simulink model "Kalman_Filter"  (R2021a)
settings: Solver=VariableStepAuto  StartTime=0.0  StopTime=10.0  RelTol=1e-3
values from neighbouring files (symbols this model uses):
  b = 2    [main_script.m]    (also in trilat2.m = dhat.^2-beacons(:,1).^2-beacons(:,2).^2)
  k1 = 0.5    [main_script.m]
  k2 = 1    [main_script.m]
  L = length(S)    [main_script.m]
  P0 = diag([0.15 0.15 deg2rad(10)].^2)    [main_script.m]
  S = [  0  100 ... (first row only)    [main_script.m]
  theta0 = 0.001    [main_script.m]
  V = eye(3)*0.01^2    [main_script.m]
  W = 10*diag([1 1 deg2rad(5)].^2)    [main_script.m]
  x0 = x0_g(1,1)+10    [main_script.m]
  y0 = x0_g(1,2)-10    [main_script.m]
libraries: simulink x5, robotcorelib x2
settings Model: Creator=csanc  LastModifiedBy=csanc

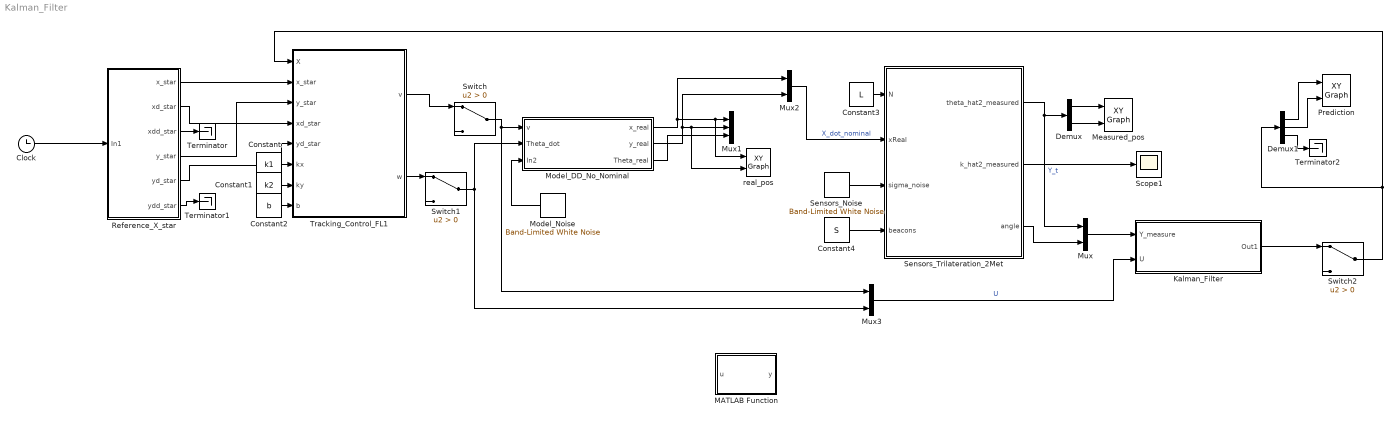
== system Kalman_Filter ==
  Clock : Clock
  Constant : Constant  Value=k1
  Constant1 : Constant  Value=k2
  Constant2 : Constant  Value=b
  Constant3 : Constant  Value=L
  Constant4 : Constant  Value=S
  Demux : Demux  Outputs=2
  Demux1 : Demux  Outputs=3
  Kalman_Filter : Subsystem
  MATLAB Function : MATLAB Function  TreatAsAtomicUnit=on
  Measured_pos : simulink/Sinks/XY Graph  xmin=0  xmax=100  ymin=0  ymax=100  st=-1
  Model_DD_No_Nominal : Subsystem
  Model_Noise : simulink/Sources/Band-Limited White Noise  Cov=[0.01]  Ts=0.05  seed=[23341]
  Mux : Mux  Inputs=2
  Mux1 : Mux  Inputs=3
  Mux2 : Mux  Inputs=2
  Mux3 : Mux  Inputs=2
  Prediction : simulink/Sinks/XY Graph  xmin=0  xmax=100  ymin=0  ymax=100  st=-1
  Reference_X_star : Subsystem
  Scope1 : Scope
  Sensors_Noise : simulink/Sources/Band-Limited White Noise  Cov=[0.05]  Ts=0.05  seed=[23341]
  Sensors_Trilateration_2Met : MATLAB Function  TreatAsAtomicUnit=on
  Switch : Switch  Criteria=u2 > Threshold
  Switch1 : Switch  Criteria=u2 > Threshold
  Switch2 : Switch  Criteria=u2 > Threshold
  Terminator : Terminator
  Terminator1 : Terminator
  Terminator2 : Terminator
  Tracking_Control_FL1 : MATLAB Function  TreatAsAtomicUnit=on
  real_pos : simulink/Sinks/XY Graph  xmin=0  xmax=105  ymin=0  ymax=105  st=-1
  wires:
  Clock/1 -> Reference_X_star/1(In1)
  Mux2/1 -> Sensors_Trilateration_2Met/2(xReal)  "X_dot_nominal"
  Constant3/1 -> Sensors_Trilateration_2Met/1(N)
  Sensors_Noise/1 -> Sensors_Trilateration_2Met/3(sigma_noise)
  Sensors_Trilateration_2Met/1(theta_hat2_measured) -> Mux/1, Demux/1  "Y_t"
  Demux/2 -> Measured_pos/2
  Constant4/1 -> Sensors_Trilateration_2Met/4(beacons)
  Demux/1 -> Measured_pos/1
  Sensors_Trilateration_2Met/2(k_hat2_measured) -> Scope1/1
  Model_DD_No_Nominal/2(y_real) -> Mux2/2, real_pos/2, Mux1/2
  Model_DD_No_Nominal/1(x_real) -> Mux2/1, real_pos/1, Mux1/1
  Model_DD_No_Nominal/3(Theta_real) -> Mux1/3
  Model_Noise/1 -> Model_DD_No_Nominal/3(In2)
  Tracking_Control_FL1/1(v) -> Switch/1
  Constant/1 -> Tracking_Control_FL1/6(kx)
  Constant1/1 -> Tracking_Control_FL1/7(ky)
  Constant2/1 -> Tracking_Control_FL1/8(b)
  Reference_X_star/1(x_star) -> Tracking_Control_FL1/2(x_star)
  Reference_X_star/4(y_star) -> Tracking_Control_FL1/3(y_star)
  Reference_X_star/2(xd_star) -> Tracking_Control_FL1/4(xd_star)
  Reference_X_star/5(yd_star) -> Tracking_Control_FL1/5(yd_star)
  Reference_X_star/3(xdd_star) -> Terminator/1
  Reference_X_star/6(ydd_star) -> Terminator1/1
  Sensors_Trilateration_2Met/3(angle) -> Mux/2
  Demux1/3 -> Terminator2/1
  Demux1/1 -> Prediction/1
  Demux1/2 -> Prediction/2
  Kalman_Filter/1(Out1) -> Switch2/1
  Mux/1 -> Kalman_Filter/1(Y_measure)
  Mux3/1 -> Kalman_Filter/2(U)  "U"
  Switch/1 -> Mux3/1, Model_DD_No_Nominal/1(v)
  Tracking_Control_FL1/2(w) -> Switch1/1
  Switch1/1 -> Model_DD_No_Nominal/2(Theta_dot), Mux3/2
  Switch2/1 -> Demux1/1, Tracking_Control_FL1/1(X)

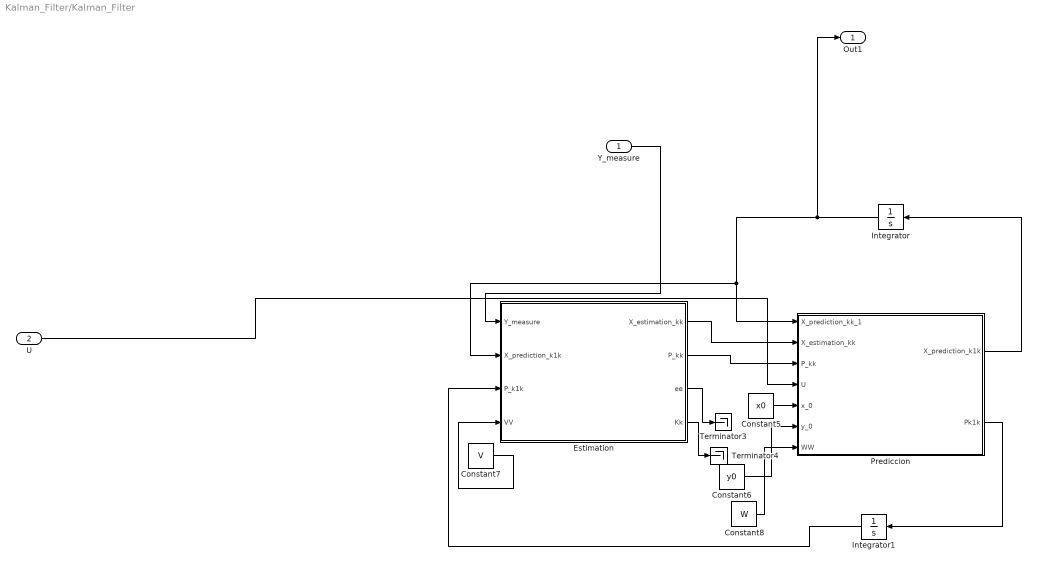
== system Kalman_Filter/Kalman_Filter ==
  Y_measure : Inport
  U : Inport  Port=2
  Constant5 : Constant  Value=x0
  Constant6 : Constant  Value=y0
  Constant7 : Constant  Value=V
  Constant8 : Constant  Value=W
  Estimation : MATLAB Function  TreatAsAtomicUnit=on
  Integrator : Integrator  InitialCondition=[x0;y0;theta0]
  Integrator1 : Integrator  InitialCondition=P0
  Prediccion : MATLAB Function  TreatAsAtomicUnit=on
  Terminator3 : Terminator
  Terminator4 : Terminator
  Out1 : Outport
  wires:
  Estimation/3(ee) -> Terminator3/1
  Integrator/1 -> Out1/1, Prediccion/1(X_prediction_kk_1), Estimation/2(X_prediction_k1k)
  Estimation/4(Kk) -> Terminator4/1
  Constant7/1 -> Estimation/4(VV)
  Constant5/1 -> Prediccion/5(x_0)
  Integrator1/1 -> Estimation/3(P_k1k)
  Y_measure/1 -> Estimation/1(Y_measure)
  Constant6/1 -> Prediccion/6(y_0)
  Prediccion/1(X_prediction_k1k) -> Integrator/1
  Prediccion/2(Pk1k) -> Integrator1/1
  Constant8/1 -> Prediccion/7(WW)
  Estimation/1(X_estimation_kk) -> Prediccion/2(X_estimation_kk)
  U/1 -> Prediccion/4(U)
  Estimation/2(P_kk) -> Prediccion/3(P_kk)

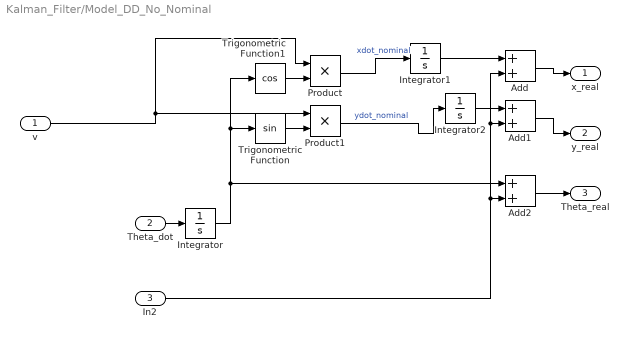
== system Kalman_Filter/Model_DD_No_Nominal ==
  v : Inport
  Theta_dot : Inport  Port=2
  In2 : Inport  Port=3
  Add : Sum
  Add1 : Sum
  Add2 : Sum
  Integrator : Integrator  InitialCondition=theta0
  Integrator1 : Integrator  InitialCondition=x0
  Integrator2 : Integrator  InitialCondition=y0
  Product : Product
  Product1 : Product
  Trigonometric Function : Trigonometry
  Trigonometric Function1 : Trigonometry  Operator=cos
  x_real : Outport
  y_real : Outport  Port=2
  Theta_real : Outport  Port=3
  wires:
  Theta_dot/1 -> Integrator/1
  Trigonometric Function/1 -> Product1/2
  Product1/1 -> Integrator2/1  "ydot_nominal"
  Trigonometric Function1/1 -> Product/2
  Integrator/1 -> Add2/1, Trigonometric Function/1, Trigonometric Function1/1
  v/1 -> Product/1, Product1/1
  Product/1 -> Integrator1/1  "xdot_nominal"
  Integrator1/1 -> Add/1
  Add/1 -> x_real/1
  Integrator2/1 -> Add1/1
  Add1/1 -> y_real/1
  Add2/1 -> Theta_real/1
  In2/1 -> Add2/2, Add1/2, Add/2

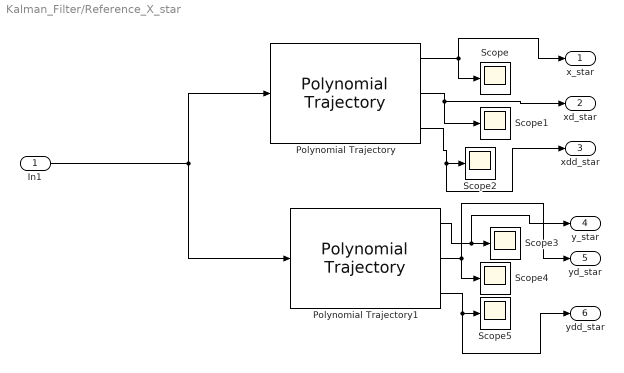
== system Kalman_Filter/Reference_X_star ==
  In1 : Inport
  Polynomial Trajectory : robotcorelib/Polynomial Trajectory  WaypointSource=Internal  Waypoints="[8.6449   70.0000   83.1776]"  TimePoints=|  TimeInterval=[ 1, 4 ]  Method=Quintic Polynomial  ParameterSource=Internal  VelocityBoundaryCondition=zeros( 1, 3 )  AccelerationBoundaryCondition=zeros( 1, 3)  SimulateUsing=Interpreted execution
      | [0    6.3867    9.9587
      | ]
  Polynomial Trajectory1 : robotcorelib/Polynomial Trajectory  WaypointSource=Internal  Waypoints="[ 37.2664   55.0000   88.2009]"  TimePoints=|  TimeInterval=[ 1, 4 ]  Method=Quintic Polynomial  ParameterSource=Internal  VelocityBoundaryCondition=zeros( 1, 3 )  AccelerationBoundaryCondition=zeros( 1, 3 )  SimulateUsing=Interpreted execution
      | [ 0    6.3867    9.9587
      | ]
  Scope{,1..5} (6 alike) : Scope
  x_star : Outport
  xd_star : Outport  Port=2
  xdd_star : Outport  Port=3
  y_star : Outport  Port=4
  yd_star : Outport  Port=5
  ydd_star : Outport  Port=6
  wires:
  Polynomial Trajectory/1 -> x_star/1, Scope/1
  Polynomial Trajectory/2 -> Scope1/1, xd_star/1
  Polynomial Trajectory/3 -> xdd_star/1, Scope2/1
  Polynomial Trajectory1/3 -> ydd_star/1, Scope5/1
  Polynomial Trajectory1/2 -> yd_star/1, Scope4/1
  In1/1 -> Polynomial Trajectory/1, Polynomial Trajectory1/1
  Polynomial Trajectory1/1 -> y_star/1, Scope3/1

== matlab function Kalman_Filter/Tracking_Control_FL1 ==
  data: v output; X input; x_star input; y_star input; xd_star input; yd_star input; kx input; ky input; b input; w output

function [v,w] = robot_control_for_No_Nominal_FL_sim(X,x_star,y_star,xd_star,yd_star,kx,ky,b)


x=X(1);
y=X(2);
theta=X(3);

xB=x+b*cos(theta);
yB=y+b*sin(theta);

xstar=x_star;
ystar=y_star;

xBdotstar=xd_star;
yBdotstar=yd_star;


Tinv=[
     cos(theta)   sin(theta);
    -sin(theta)/b cos(theta)/b
    ];
ux=xBdotstar+kx*(xstar-xB);
uy=yBdotstar+ky*(ystar-yB);

vw=Tinv*[ux;uy];
v=vw(1);
w=vw(2);
% Xdot=[
%     v*cos(theta);
%     v*sin(theta);
%     w
%     ];

end

== matlab function Kalman_Filter/Estimation ==
  data: Y_measure input; X_estimation_kk output; X_prediction_k1k input; P_kk output; ee output; Kk output; P_k1k input; VV input
function[X_estimation_kk,P_kk,ee,Kk]=Kalman_Filter(Y_measure,X_prediction_k1k,P_k1k,VV)
Ck=[1 0 0;
    0 1 0
    0 0 1];

%% kalman gain
Kk=P_k1k*Ck'*inv(((Ck*P_k1k*Ck'+VV)));
 %% predicted output
 yhk=Ck*X_prediction_k1k;
%% innovation
ee=Y_measure-yhk;
%% from prediction to estimation
 X_estimation_kk=X_prediction_k1k+Kk*ee;
 P_kk=P_k1k-Kk*Ck*P_k1k;

== matlab function Kalman_Filter/Sensors_Trilateration_2Met ==
  data: N input; theta_hat2_measured output; xReal input; sigma_noise input; beacons input; k_hat2_measured output; angle output
function [theta_hat2_measured,k_hat2_measured, angle] = trilateration_second_method(N,xReal,sigma_noise,beacons)
 
f=@(theta,beacons)(sqrt((beacons(:,1)-theta(1)).^2+(beacons(:,2)-theta(2)).^2));
%%
%theta0=xReal+sigma_0*randn(2,1); % theta=x0,y0
%%
d=f(xReal,beacons);%distancia entre beacons y medida real
dhat=d+sigma_noise;% distancia con noise de sensor
% % %% tecnica 1
% % J=zeros(N,2);
% % for k=1:N %% N numero de beacons
% %     xc=beacons(k,1)
% %     yc=beacons(k,2)
% %     dc=norm(beacons(k,:)-theta0(:)');
% %     Jx=(theta0(1)-xc)/dc;
% %     Jy=(theta0(2)-yc)/dc;
% %      J(k,:)=[Jx Jy];
% %  end
% %  theta_hat1=theta0+pinv(J)*(dhat-f(theta0,beacons));
% %  [theta_hat1]=trilat1(beacons,dhat,theta0);
%% tecnica 2
[theta_hat2_measured,k_hat2_measured,angle]=trilat2(beacons,dhat);
%% tecnica 3
% [theta_hat3]=trilat3(beacons,dhat);
%% Si hay como dibubar pero se debe arreglar 
% % % figure();hold on;grid on;
% % % plot(beacons(:,1),beacons(:,2),'ok','LineWidth',3);axis('equal');
% % % for k=1:length(d)
% % %     alpha=atan2(beacons(k,2)-xReal(2),beacons(k,1)-xReal(1));
% % %     alpha1=atan2(-beacons(k,2)+xReal(2),-beacons(k,1)+xReal(1));
% % %     line([xReal(1) xReal(1)+d(k)*cos(alpha)],[xReal(2) xReal(2)+d(k)*sin(alpha)],'Color','m','LineWidth',2);
% % %     line([beacons(k,1) beacons(k,1)+dhat(k)*cos(alpha1)],[beacons(k,2) beacons(k,2)+dhat(k)*sin(alpha1)],'Color','k','LineWidth',2,'LineStyle','--');
% % % end
%plot(xReal(1),xReal(2),'xb','LineWidth',3);
%plot(theta_hat1(1),theta_hat1(2),'om','LineWidth',3);
%plot(theta_hat2_measured(1),theta_hat2_measured(2),'or','LineWidth',3);
%plot(theta_hat3(1),theta_hat3(2),'ok','LineWidth',3);
%norm(xReal-theta_hat1)
norm(xReal-theta_hat2_measured)
%norm(xReal-theta_hat3)

== matlab function Kalman_Filter/Prediccion ==
  data: X_prediction_kk_1 input; X_estimation_kk input; X_prediction_k1k output; P_kk input; Pk1k output; U input; x_0 input; y_0 input; WW input
function[X_prediction_k1k, Pk1k]=Kalman_Predictor(X_prediction_kk_1,X_estimation_kk,P_kk,U,x_0,y_0,WW)

theta=atan(X_estimation_kk(2)/X_estimation_kk(1));
A_t=[
    1 0 -U(1)*sin(theta);
    0 1  U(1)*cos(theta);
    0 0             1
    ];
%% from estimation to prediction
X_prediction_k1k=[U(1)*cos(X_prediction_kk_1(3));
    U(1)*sin(X_prediction_kk_1(3));
    U(2)];
Pk1k=A_t.*P_kk.*A_t'+WW;

end

== matlab function Kalman_Filter/MATLAB Function ==
  data: u input; y output
function y = fcn(u)

y = u;
